simulink model "mult35x35_tb"  (Simulink 6.6)
settings: Solver=ode45  StartTime=0.0  StopTime=1000  RelTol=1e-3
undefined symbols (not defined in the file): A, B
libraries: xbsIndex_r4 x168, simulink x2, xbsCopyrightNotice_r4 x1
(part 1 of 2)
settings Model: Creator=singhj  LastModifiedBy=juttu
settings DataIOCC: SignalLoggingName=sigsOut
settings OptimizationCC: InlineInvariantSignals=on
settings DebuggingCC: SignalResolutionControl=TryResolveAllWithWarning  SolverPrmCheckMsg=none  MultiTaskDSMMsg=warning  MultiTaskCondExecSysMsg=none  StrictBusMsg=None
settings HardwareCC: TargetUnknown=on
settings RTWCC: IncludeERTFirstTime=on

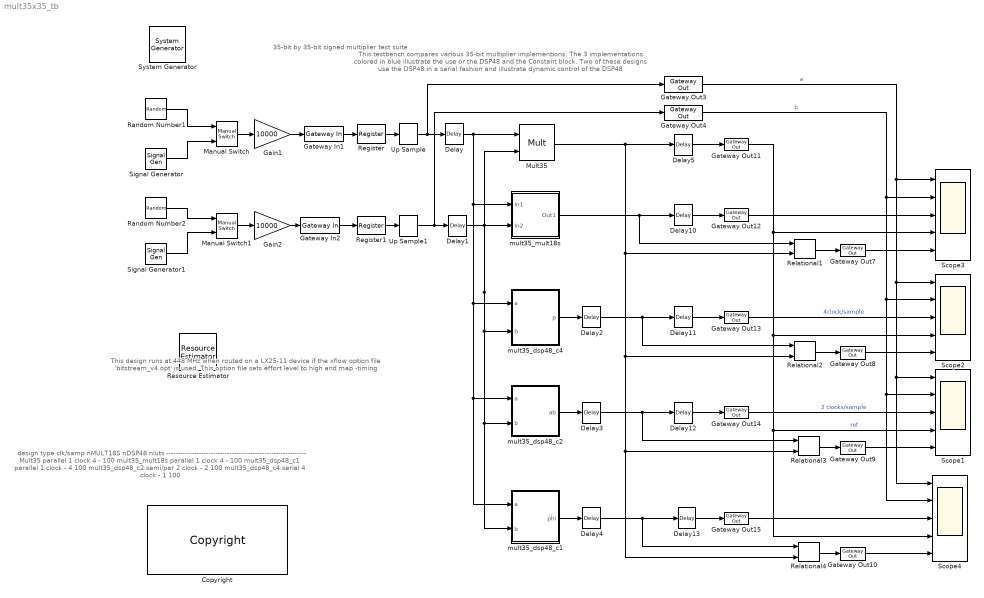
== system mult35x35_tb ==
  note: 35-bit by 35-bit signed multiplier test suite
  note: This testbench compares various 35-bit multiplier implementions.
      | The 3 implementations colored in blue illustrate the use or the DSP48
      | and the Constant block. Two of these designs use the DSP48 in a serial
      | fashion and illustrate dynamic control of the DSP48
  note: design           type       clk/samp  nMULT18S nDSP48 nluts
      | ------------------------------------------------------------
      | Mult35           parallel   1 clock     4       -      100
      | mult35_mult18s   parallel   1 clock     4       -      100
      | mult35_dsp48_c1  parallel   1 clock     -       4      100
      | mult35_dsp48_c2  semi/par   2 clock     -       2      100
      | mult35_dsp48_c4  serial     4 clock     -       1      100
  note: This design runs at 448 MHz
      | when routed on a LX25-11 device if the
      | xflow option file 'bitstream_v4.opt' is used.
      | This option file sets effort level to high
      | and map -timing
  " System Generator" : xbsIndex_r4/ System Generator  Tag=genX  SystemSampleTime=-1  xilinxfamily=Virtex4  part=xc4vlx25  speed=-11  package=ff668  synthesis_tool=Synplify Pro  clock_wrapper=Clock Enables  directory=./netlist  testbench=off  simulink_period=1  sysclk_period=100  dcm_input_clock_period=100  incr_netlist=off  trim_vbits=Everywhere in SubSystem  dbl_ovrd=According to Block Masks  core_generation=According to Block Masks  run_coregen=off  deprecated_control=off  eval_field=0  block_type=sysgen
      settings: block_version=8.2.EA1
  Copyright : xbsCopyrightNotice_r4/Copyright  block_type=copyright
      settings: block_version=10.1.00
      settings: infoedit=|
      | Copyright(C) 2008 by  Xilinx, Inc. All rights reserved.<br>
      | <br>
      | This file contains proprietary, confidential information of Xilinx, Inc., is distributed under license
      | from Xilinx, Inc., and may be used, copied and/or disclosed only pursuant to the terms of a valid license
      | agreement with Xilinx, Inc. Xilinx hereby grants you a license to use this file solely for design,
      | simulation, implementation and creation of design files limited to Xilinx devices or technologies. Use
      | with non-Xilinx devices or technologies is expressly prohibited and immediately terminates your license
      | unless covered by a separate agreement.<br>
      | <br>
      | Xilinx is providing this design, code, or information "as-is" solely for use in developing programs and
      | solutions for Xilinx devices, with no obligation on the part of Xilinx to provide support. By providing
      | this design, code, or information as one possible implementation of this feature, application or standard,
      | Xilinx is making no representation that this implementation is free from any claims of infringement. You
      | are responsible for obtaining any rights you may require for your implementation. Xilinx expressly disclaims
      | any warranty whatsoever with respect to the adequacy of the implementation, including but not limited to any
      | warranties or representations that this implementation is free from claims of infringement, implied warranties
      | of merchantability or fitness for a particular purpose.<br>
      | <br>
      | Xilinx products are not intended for use in life support appliances, devices, or systems. Use in such
      | applications is expressly prohibited.<br>
      | <br>
      | Any modifications that are made to the Source Code are done at the user's sole risk and will be unsupported.<br>
      | <br>
      | This copyright and support notice must be retained as part of this text at all times.
      | (c) Copyright 1995-2008 Xilinx, Inc. All rights reserved.
  Delay{,1..4} (5 alike) : xbsIndex_r4/Delay  en=off  latency=3  dbl_ovrd=off  reg_retiming=on  block_type=delay
      settings: infoedit="Delay line having  configurable length.<P><P>Hardware notes: A delay line is a chain, each link of which is an SRL16 followed by a flip-flop. If register retiming is enabled, the delay line is a chain of flip-flops."  xl_area=[0, 0, 0, 0, 0, 0, 0]  block_version=VER_STRING_GOES_HERE
  Delay10 : xbsIndex_r4/Delay  en=off  latency=15  dbl_ovrd=off  reg_retiming=on  block_type=delay
      settings: infoedit="Delay line having  configurable length.<P><P>Hardware notes: A delay line is a chain, each link of which is an SRL16 followed by a flip-flop. If register retiming is enabled, the delay line is a chain of flip-flops."  xl_area=[0, 0, 0, 0, 0, 0, 0]  block_version=VER_STRING_GOES_HERE
  Delay11 : xbsIndex_r4/Delay  en=off  latency=5  dbl_ovrd=off  reg_retiming=on  block_type=delay
      settings: infoedit="Delay line having  configurable length.<P><P>Hardware notes: A delay line is a chain, each link of which is an SRL16 followed by a flip-flop. If register retiming is enabled, the delay line is a chain of flip-flops."  xl_area=[0, 0, 0, 0, 0, 0, 0]  block_version=VER_STRING_GOES_HERE
  Delay12 : xbsIndex_r4/Delay  en=off  latency=6  dbl_ovrd=off  reg_retiming=on  block_type=delay
      settings: infoedit="Delay line having  configurable length.<P><P>Hardware notes: A delay line is a chain, each link of which is an SRL16 followed by a flip-flop. If register retiming is enabled, the delay line is a chain of flip-flops."  xl_area=[0, 0, 0, 0, 0, 0, 0]  block_version=VER_STRING_GOES_HERE
  Delay13 : xbsIndex_r4/Delay  en=off  latency=9  dbl_ovrd=off  reg_retiming=on  block_type=delay
      settings: infoedit="Delay line having  configurable length.<P><P>Hardware notes: A delay line is a chain, each link of which is an SRL16 followed by a flip-flop. If register retiming is enabled, the delay line is a chain of flip-flops."  xl_area=[0, 0, 0, 0, 0, 0, 0]  block_version=VER_STRING_GOES_HERE
  Delay5 : xbsIndex_r4/Delay  en=off  latency=13  dbl_ovrd=off  reg_retiming=on  block_type=delay
      settings: infoedit="Delay line having  configurable length.<P><P>Hardware notes: A delay line is a chain, each link of which is an SRL16 followed by a flip-flop. If register retiming is enabled, the delay line is a chain of flip-flops."  xl_area=[0, 0, 0, 0, 0, 0, 0]  block_version=VER_STRING_GOES_HERE
  Gain1 : Gain  Gain=10000  SampleTime=4  SaturateOnIntegerOverflow=on
  Gain2 : Gain  Gain=10000  SampleTime=4  SaturateOnIntegerOverflow=on
  Gateway In1 : xbsIndex_r4/Gateway In  arith_type="Signed  (2's comp)"  n_bits=35  bin_pt=0  quantization="Round  (unbiased: +/- Inf)"  overflow=Saturate  period=4  dbl_ovrd=off  timing_constraint=None  locs_specified=off  LOCs={}  block_type=gatewayin
      settings: infoedit="Gateway in block.  Converts inputs of type Simulink integer, double and fixed point to  Xilinx fixed point type.<P><P>Hardware notes:  In hardware these blocks become top level input ports."  xl_area=[0 0 0 0 35 0 0]  block_version=VER_STRING_GOES_HERE
  Gateway In2 : xbsIndex_r4/Gateway In  arith_type="Signed  (2's comp)"  n_bits=35  bin_pt=0  quantization="Round  (unbiased: +/- Inf)"  overflow=Saturate  period=4  dbl_ovrd=off  timing_constraint=None  locs_specified=off  LOCs={}  block_type=gatewayin
      settings: infoedit="Gateway in block.  Converts inputs of type Simulink integer, double and fixed point to  Xilinx fixed point type.<P><P>Hardware notes:  In hardware these blocks become top level input ports."  xl_area=[0 0 0 0 35 0 0]  block_version=VER_STRING_GOES_HERE
  Gateway Out{7..15} (9 alike) : xbsIndex_r4/Gateway Out  hdl_port=on  timing_constraint=None  locs_specified=off  LOCs={}  block_type=gatewayout
      settings: infoedit="Gateway out block.  Converts Xilinx fixed point inputs into ouputs of type Simulink integer, double, or fixed point.<P><P>Hardware notes:  In hardware these blocks become top level output ports or are discarded, depending on how they are configured."  xl_area=[0 0 0 0 70 0 0]  block_version=VER_STRING_GOES_HERE
  Gateway Out3 : xbsIndex_r4/Gateway Out  hdl_port=off  timing_constraint=None  locs_specified=off  LOCs={}  block_type=gatewayout
      settings: infoedit="Gateway out block.  Converts Xilinx fixed point inputs into ouputs of type Simulink integer, double, or fixed point.<P><P>Hardware notes:  In hardware these blocks become top level output ports or are discarded, depending on how they are configured."  xl_area=[0 0 0 0 70 0 0]  block_version=VER_STRING_GOES_HERE
  Gateway Out4 : xbsIndex_r4/Gateway Out  hdl_port=off  timing_constraint=None  locs_specified=off  LOCs={}  block_type=gatewayout
      settings: infoedit="Gateway out block.  Converts Xilinx fixed point inputs into ouputs of type Simulink integer, double, or fixed point.<P><P>Hardware notes:  In hardware these blocks become top level output ports or are discarded, depending on how they are configured."  xl_area=[0 0 0 0 70 0 0]  block_version=VER_STRING_GOES_HERE
  Manual Switch : simulink/Signal Routing/Manual Switch  SystemSampleTime=-1  sw=0  action=0  varsize=off
  Manual Switch1 : simulink/Signal Routing/Manual Switch  SystemSampleTime=-1  sw=0  action=0  varsize=off
  Mult35 : xbsIndex_r4/Mult  precision=Full  arith_type="Signed  (2's comp)"  n_bits=8  bin_pt=2  quantization=Truncate  overflow=Wrap  en=off  latency=5  dbl_ovrd=off  use_behavioral_HDL=off  use_embedded=on  opt=Speed  optimum_pipeline=off  pipeline=on  use_rpm=on  placement_style=Rectangular shape  block_type=mult
      settings: infoedit=Multiplies two values.<P><P>Hardware notes: To use the internal pipeline stage of the dedicated multiplier you must select 'Pipeline to Greatest Extent Possible'.  xl_area=[231 460 0 269 0 4 0]  block_version=VER_STRING_GOES_HERE
  Random Number1 : RandomNumber  SampleTime=0
  Random Number2 : RandomNumber  SampleTime=0
  Register : xbsIndex_r4/Register  init=0  rst=off  en=off  dbl_ovrd=off  block_type=register
      settings: block_version=VER_STRING_GOES_HERE
  Register1 : xbsIndex_r4/Register  init=0  rst=off  en=off  dbl_ovrd=off  block_type=register
      settings: block_version=VER_STRING_GOES_HERE
  Relational{1..4} (4 alike) : xbsIndex_r4/Relational  mode=a!=b  en=off  latency=1  dbl_ovrd=off  block_type=relational
      settings: block_version=10.1.2-Beta
  Resource Estimator : xbsIndex_r4/Resource Estimator  Tag=resEstTag  Slices=896  FFs=1554  BRAMs=0  LUTs=775  IOBs=545  EBMs=8  TBUFs=0  xl_use_estimator_area=off  est_options=Estimate  xl_estimator_area=[896 1554 0 775 545 8 0]  mrp_directory=C:/1proj/designs/firs/fir_t1_pipe/par_v1_g1  simulink_period=1/16  block_type=resource_estimator
      settings: AttributesFormatString=Resource\nEstimator  block_version=8.2.EA1
  Scope{1..4} (4 alike) : Scope  NumInputPorts=5
      Scope1 settings: TimeRange=100  YMin=-100~-100~0~0~-1  YMax=100~100~10000~10000~1
      Scope2 settings: TimeRange=100  YMin=-100~-100~0~0~-1  YMax=100~100~10000~10000~1  SaveName=ScopeData3
      Scope3 settings: TimeRange=100  YMin=-100~-100~0~0~-1  YMax=100~100~10000~10000~1  SaveName=ScopeData4
      Scope4 settings: TimeRange=100  YMin=-100~-100~0~0~-1  YMax=100~100~10000~10000~1  SaveName=ScopeData5
  Signal Generator : SignalGenerator  Amplitude=100  Frequency=.00300
  Signal Generator1 : SignalGenerator  Amplitude=100  Frequency=.0200
  Up Sample : xbsIndex_r4/Up Sample  sample_ratio=4  copy_samples=on  dbl_ovrd=off  block_type=usamp
      settings: infoedit="Up samples input data.  Inserted values  can be zeros or copies of the most recent input sample.<P><P>Hardware notes: No hardware is needed if inserted values are copies of the input sample; otherwise, a mux and single bit flip-flop are used."  xl_area=[0, 0, 0, 0, 0, 0, 0]  block_version=VER_STRING_GOES_HERE
  Up Sample1 : xbsIndex_r4/Up Sample  sample_ratio=4  copy_samples=on  dbl_ovrd=off  block_type=usamp
      settings: infoedit="Up samples input data.  Inserted values  can be zeros or copies of the most recent input sample.<P><P>Hardware notes: No hardware is needed if inserted values are copies of the input sample; otherwise, a mux and single bit flip-flop are used."  xl_area=[0, 0, 0, 0, 0, 0, 0]  block_version=VER_STRING_GOES_HERE
  mult35_dsp48_c1 : Subsystem
  mult35_dsp48_c2 : Subsystem
  mult35_dsp48_c4 : Subsystem
  mult35_mult18s : Subsystem
  wires:
  Mult35/1 -> Relational1/2, Relational2/2, Relational3/2, Relational4/2, Delay5/1
  mult35_dsp48_c4/1(p) -> Delay2/1
  mult35_mult18s/1(Out1) -> Relational1/1, Delay10/1
  Signal Generator/1 -> Manual Switch/2
  mult35_dsp48_c2/1(ab) -> Delay3/1
  mult35_dsp48_c1/1(phi) -> Delay4/1
  Random Number1/1 -> Manual Switch/1
  Manual Switch/1 -> Gain1/1
  Gain1/1 -> Gateway In1/1
  Signal Generator1/1 -> Manual Switch1/2
  Random Number2/1 -> Manual Switch1/1
  Manual Switch1/1 -> Gain2/1
  Gateway In1/1 -> Register/1
  Gateway In2/1 -> Register1/1
  Gateway Out11/1 -> Scope3/4, Scope2/4, Scope1/4, Scope4/4  "ref"
  Gateway Out14/1 -> Scope1/3  "2 clocks/sample"
  Gateway Out13/1 -> Scope2/3  "4clock/sample"
  Gateway Out12/1 -> Scope3/3
  Gain2/1 -> Gateway In2/1
  Delay/1 -> mult35_dsp48_c1/1(a), mult35_dsp48_c2/1(a), mult35_dsp48_c4/1(a), mult35_mult18s/1(In1), Mult35/1
  Delay1/1 -> mult35_dsp48_c1/2(b), mult35_dsp48_c2/2(b), mult35_dsp48_c4/2(b), mult35_mult18s/2(In2), Mult35/2
  Delay2/1 -> Relational2/1, Delay11/1
  Delay3/1 -> Relational3/1, Delay12/1
  Delay4/1 -> Relational4/1, Delay13/1
  Up Sample/1 -> Delay/1, Gateway Out3/1
  Up Sample1/1 -> Delay1/1, Gateway Out4/1
  Gateway Out3/1 -> Scope3/1, Scope2/1, Scope4/1, Scope1/1  "a"
  Gateway Out4/1 -> Scope4/2, Scope1/2, Scope2/2, Scope3/2  "b"
  Gateway Out15/1 -> Scope4/3
  Register/1 -> Up Sample/1
  Register1/1 -> Up Sample1/1
  Relational1/1 -> Gateway Out7/1
  Gateway Out8/1 -> Scope2/5
  Gateway Out9/1 -> Scope1/5
  Gateway Out7/1 -> Scope3/5
  Relational2/1 -> Gateway Out8/1
  Relational3/1 -> Gateway Out9/1
  Relational4/1 -> Gateway Out10/1
  Gateway Out10/1 -> Scope4/5
  Delay5/1 -> Gateway Out11/1
  Delay10/1 -> Gateway Out12/1
  Delay11/1 -> Gateway Out13/1
  Delay12/1 -> Gateway Out14/1
  Delay13/1 -> Gateway Out15/1

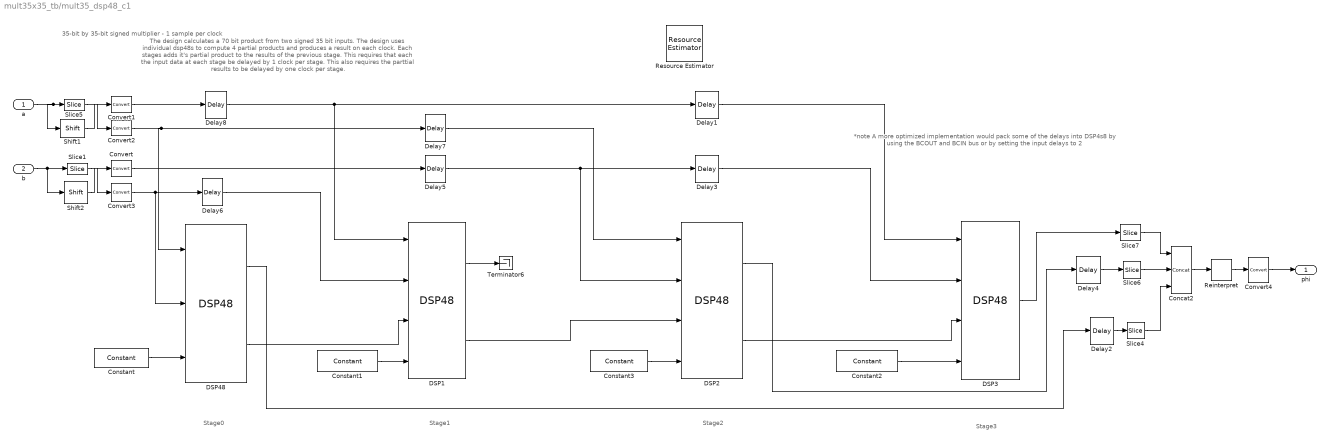
== system mult35x35_tb/mult35_dsp48_c1 ==
  note: The design calculates a 70 bit product from two signed 35 bit inputs.
      | The design uses individual dsp48s to compute 4 partial products and produces a result on each clock.
      | Each stages adds it's partial product to the results of the previous stage. This requires that each the
      | input data at each stage be delayed by 1 clock per stage. This also requires the parttial results to be delayed
      | by one clock per stage.
  note: 35-bit by 35-bit signed multiplier -
      | 1 sample per clock
  note: *note
      | A more optimized implementation
      | would pack some of the delays into
      | DSP4s8 by using the BCOUT and BCIN
      |  bus or  by setting the input delays to 2
  note: Stage3
  note: Stage2
  note: Stage1
  note: Stage0
  a : Inport
  b : Inport  Port=2
  Concat2 : xbsIndex_r4/Concat  num_inputs=3  dbl_ovrd=off  block_type=concat
      settings: block_version=VER_STRING_GOES_HERE
  Constant : xbsIndex_r4/Constant  arith_type=DSP48 Instruction  const=1  n_bits=1  bin_pt=0  explicit_period=off  period=1  equ=P=+A*B  opselect=A * B  inp2=PCIN>>17  opr=+  inp1=P  carry=CIN  dbl_ovrd=off  block_type=constant
      settings: block_version=VER_STRING_GOES_HERE
  Constant1 : xbsIndex_r4/Constant  arith_type=DSP48 Instruction  const=1  n_bits=1  bin_pt=0  explicit_period=off  period=1  equ=P=PCIN>>17+(A*B)  opselect=Custom  inp2=PCIN>>17  opr=+  inp1=A*B  carry=0  dbl_ovrd=off  block_type=constant
      settings: block_version=VER_STRING_GOES_HERE
  Constant2 : xbsIndex_r4/Constant  arith_type=DSP48 Instruction  const=1  n_bits=1  bin_pt=0  explicit_period=off  period=1  equ=P=PCIN>>17+(A*B)  opselect=Custom  inp2=PCIN>>17  opr=+  inp1=A*B  carry=0  dbl_ovrd=off  block_type=constant
      settings: block_version=VER_STRING_GOES_HERE
  Constant3 : xbsIndex_r4/Constant  arith_type=DSP48 Instruction  const=1  n_bits=1  bin_pt=0  explicit_period=off  period=1  equ=P=PCIN+(A*B)  opselect=Custom  inp2=PCIN  opr=+  inp1=A*B  carry=0  dbl_ovrd=off  block_type=constant
      settings: block_version=VER_STRING_GOES_HERE
  Convert{,1..3} (4 alike) : xbsIndex_r4/Convert  arith_type="Signed  (2's comp)"  n_bits=18  bin_pt=0  quantization=Truncate  overflow=Wrap  latency=0  dbl_ovrd=off  pipeline=off  block_type=convert
      settings: infoedit=The input is presented at the output after quantization and overflow effects.<P><P>Hardware notes: Additional hardware is used when rounding or saturation is selected and output width is less than the input width.  xl_area=[0 0 0 0 0 0 0]  block_version=VER_STRING_GOES_HERE
  Convert4 : xbsIndex_r4/Convert  arith_type="Signed  (2's comp)"  n_bits=71  bin_pt=0  quantization=Truncate  overflow=Wrap  latency=0  dbl_ovrd=off  pipeline=off  block_type=convert
      settings: infoedit=The input is presented at the output after quantization and overflow effects.<P><P>Hardware notes: Additional hardware is used when rounding or saturation is selected and output width is less than the input width.  xl_area=[0 0 0 0 0 0 0]  block_version=VER_STRING_GOES_HERE
  DSP1 : xbsIndex_r4/DSP48  use_b=Direct from B Port  use_op=on  use_creg=off  use_pcin=on  use_pcout=on  use_bcout=off  rst_all=off  en_all=off  pipeline_a=1  pipeline_b=1  pipeline_c=on  pipeline_p=on  pipeline_mult=on  pipeline_opmode=on  pipeline_sub=on  pipeline_carryin=on  pipeline_carryinsel=on  rst_a=off  rst_b=off  rst_c=off  rst_mult=off  rst_p=off  rst_carry_in=off  rst_ctrl=off  en_a=off  en_b=off  en_c=off  en_mult=off  en_p=off  en_carry_in=off  en_ctrl=off  dbl_ovrd=off  use_synth_model=off  xl_useadderonly=off  block_type=dsp48
      settings: xl_use_area=on  xl_area=[0, 0, 0, 0, 0, 0, 0]  block_version=VER_STRING_GOES_HERE
  DSP2 : xbsIndex_r4/DSP48  use_b=Direct from B Port  use_op=on  use_creg=off  use_pcin=on  use_pcout=on  use_bcout=off  rst_all=off  en_all=off  pipeline_a=1  pipeline_b=1  pipeline_c=on  pipeline_p=on  pipeline_mult=on  pipeline_opmode=on  pipeline_sub=on  pipeline_carryin=on  pipeline_carryinsel=on  rst_a=off  rst_b=off  rst_c=off  rst_mult=off  rst_p=off  rst_carry_in=off  rst_ctrl=off  en_a=off  en_b=off  en_c=off  en_mult=off  en_p=off  en_carry_in=off  en_ctrl=off  dbl_ovrd=off  use_synth_model=off  xl_useadderonly=off  block_type=dsp48
      settings: xl_use_area=on  xl_area=[0, 0, 0, 0, 0, 0, 0]  block_version=VER_STRING_GOES_HERE
  DSP3 : xbsIndex_r4/DSP48  use_b=Direct from B Port  use_op=on  use_creg=off  use_pcin=on  use_pcout=off  use_bcout=off  rst_all=off  en_all=off  pipeline_a=1  pipeline_b=1  pipeline_c=on  pipeline_p=on  pipeline_mult=on  pipeline_opmode=on  pipeline_sub=on  pipeline_carryin=on  pipeline_carryinsel=on  rst_a=off  rst_b=off  rst_c=off  rst_mult=off  rst_p=off  rst_carry_in=off  rst_ctrl=off  en_a=off  en_b=off  en_c=off  en_mult=off  en_p=off  en_carry_in=off  en_ctrl=off  dbl_ovrd=off  use_synth_model=off  xl_useadderonly=off  block_type=dsp48
      settings: xl_use_area=on  xl_area=[0, 0, 0, 0, 0, 0, 0]  block_version=VER_STRING_GOES_HERE
  DSP48 : xbsIndex_r4/DSP48  use_b=Direct from B Port  use_op=on  use_creg=off  use_pcin=off  use_pcout=on  use_bcout=off  rst_all=off  en_all=off  pipeline_a=1  pipeline_b=1  pipeline_c=on  pipeline_p=on  pipeline_mult=on  pipeline_opmode=on  pipeline_sub=on  pipeline_carryin=on  pipeline_carryinsel=on  rst_a=off  rst_b=off  rst_c=off  rst_mult=off  rst_p=off  rst_carry_in=off  rst_ctrl=off  en_a=off  en_b=off  en_c=off  en_mult=off  en_p=off  en_carry_in=off  en_ctrl=off  dbl_ovrd=off  use_synth_model=off  xl_useadderonly=off  block_type=dsp48
      settings: xl_use_area=on  xl_area=[0, 0, 0, 0, 0, 0, 0]  block_version=VER_STRING_GOES_HERE
  Delay1 : xbsIndex_r4/Delay  en=off  latency=2  dbl_ovrd=off  reg_retiming=off  block_type=delay
      settings: infoedit="Delay line having  configurable length.<P><P>Hardware notes: A delay line is a chain, each link of which is an SRL16 followed by a flip-flop. If register retiming is enabled, the delay line is a chain of flip-flops."  xl_area=[9 18 0 18 0 0 0]  block_version=VER_STRING_GOES_HERE
  Delay2 : xbsIndex_r4/Delay  en=off  latency=3  dbl_ovrd=off  reg_retiming=off  block_type=delay
      settings: infoedit="Delay line having  configurable length.<P><P>Hardware notes: A delay line is a chain, each link of which is an SRL16 followed by a flip-flop. If register retiming is enabled, the delay line is a chain of flip-flops."  xl_area=[24 48 0 48 0 0 0]  block_version=VER_STRING_GOES_HERE
  Delay{3..4,6,8} (4 alike) : xbsIndex_r4/Delay  en=off  latency=1  dbl_ovrd=off  reg_retiming=off  block_type=delay
      Delay3 settings: infoedit="Delay line having  configurable length.<P><P>Hardware notes: A delay line is a chain, each link of which is an SRL16 followed by a flip-flop. If register retiming is enabled, the delay line is a chain of flip-flops."  xl_area=[9 18 0 0 0 0 0]  block_version=VER_STRING_GOES_HERE
      Delay4 settings: infoedit="Delay line having  configurable length.<P><P>Hardware notes: A delay line is a chain, each link of which is an SRL16 followed by a flip-flop. If register retiming is enabled, the delay line is a chain of flip-flops."  xl_area=[24 48 0 0 0 0 0]  block_version=VER_STRING_GOES_HERE
      Delay6 settings: infoedit="Delay line having  configurable length.<P><P>Hardware notes: A delay line is a chain, each link of which is an SRL16 followed by a flip-flop. If register retiming is enabled, the delay line is a chain of flip-flops."  xl_area=[9 18 0 0 0 0 0]  block_version=VER_STRING_GOES_HERE
      Delay8 settings: infoedit="Delay line having  configurable length.<P><P>Hardware notes: A delay line is a chain, each link of which is an SRL16 followed by a flip-flop. If register retiming is enabled, the delay line is a chain of flip-flops."  xl_area=[9 18 0 0 0 0 0]  block_version=VER_STRING_GOES_HERE
  Delay5 : xbsIndex_r4/Delay  en=off  latency=2  dbl_ovrd=off  reg_retiming=off  block_type=delay
      settings: infoedit="Delay line having  configurable length.<P><P>Hardware notes: A delay line is a chain, each link of which is an SRL16 followed by a flip-flop. If register retiming is enabled, the delay line is a chain of flip-flops."  xl_area=[9 18 0 18 0 0 0]  block_version=VER_STRING_GOES_HERE
  Delay7 : xbsIndex_r4/Delay  en=off  latency=2  dbl_ovrd=off  reg_retiming=off  block_type=delay
      settings: infoedit="Delay line having  configurable length.<P><P>Hardware notes: A delay line is a chain, each link of which is an SRL16 followed by a flip-flop. If register retiming is enabled, the delay line is a chain of flip-flops."  xl_area=[9 18 0 18 0 0 0]  block_version=VER_STRING_GOES_HERE
  Reinterpret : xbsIndex_r4/Reinterpret  force_arith_type=on  arith_type="Signed  (2's comp)"  force_bin_pt=on  bin_pt=0  block_type=cast
      settings: infoedit="Changes type of samples without altering their binary representation.<P><P>Hardware notes: In hardware this block costs nothing.<P><P>Example:  Suppose the input is 6 bits wide, signed, with 2 fractional bits, and the output is forced to unsigned with 0 fractional bits.  Then an input of -2.0 (1110.00 in binary 2's complement) becomes an output of 56 (111000 in binary)."  block_version=VER_STRING_GOES_HERE
  Resource Estimator : xbsIndex_r4/Resource Estimator  Tag=resEstTag  Slices=102  FFs=204  BRAMs=0  LUTs=102  IOBs=0  EBMs=0  TBUFs=0  xl_use_estimator_area=off  est_options=Estimate  xl_estimator_area=[102 204 0 102 0 0 0]  mrp_directory=I:\sg48\src  simulink_period=1/16  block_type=resource_estimator
      settings: AttributesFormatString=Resource\nEstimator  block_version=9.2.00
  Shift1 : xbsIndex_r4/Shift  shift_dir=Right  shift_bits=17  en=off  latency=0  precision=Full  arith_type="Signed  (2's comp)"  n_bits=8  bin_pt=2  quantization=Truncate  overflow=Wrap  dbl_ovrd=off  block_type=shift
      settings: xl_area=[0 0 0 0 0 0 0]  block_version=VER_STRING_GOES_HERE
  Shift2 : xbsIndex_r4/Shift  shift_dir=Right  shift_bits=17  en=off  latency=0  precision=Full  arith_type="Signed  (2's comp)"  n_bits=8  bin_pt=2  quantization=Truncate  overflow=Wrap  dbl_ovrd=off  block_type=shift
      settings: xl_area=[0 0 0 0 0 0 0]  block_version=VER_STRING_GOES_HERE
  Slice{1,4..6} (4 alike) : xbsIndex_r4/Slice  nbits=17  boolean_output=off  mode=Lower Bit Location + Width  bit1=18  base1=LSB of Input  bit0=0  base0=LSB of Input  dbl_ovrd=off  block_type=slice
      settings: infoedit="Extracts a given range of bits from each input sample and presents it at the output.  The output type is ordinarily unsigned with binary point at zero, but can be Boolean when the slice is one bit wide.<P><P>Hardware notes: In hardware this block costs nothing."  block_version=VER_STRING_GOES_HERE
  Slice7 : xbsIndex_r4/Slice  nbits=36  boolean_output=off  mode=Lower Bit Location + Width  bit1=18  base1=LSB of Input  bit0=0  base0=LSB of Input  dbl_ovrd=off  block_type=slice
      settings: infoedit="Extracts a given range of bits from each input sample and presents it at the output.  The output type is ordinarily unsigned with binary point at zero, but can be Boolean when the slice is one bit wide.<P><P>Hardware notes: In hardware this block costs nothing."  block_version=VER_STRING_GOES_HERE
  Terminator6 : Terminator
  phi : Outport
  wires:
  Convert4/1 -> phi/1
  Slice4/1 -> Concat2/3
  Slice6/1 -> Concat2/2
  Delay2/1 -> Slice4/1
  Slice7/1 -> Concat2/1
  Delay4/1 -> Slice6/1
  DSP3/1 -> Slice7/1
  Reinterpret/1 -> Convert4/1
  Concat2/1 -> Reinterpret/1
  Convert3/1 -> Delay6/1, DSP48/2
  Convert/1 -> Delay5/1
  Convert2/1 -> Delay7/1, DSP48/1
  Convert1/1 -> Delay8/1
  Delay1/1 -> DSP3/1
  Delay3/1 -> DSP3/2
  Delay7/1 -> DSP2/1
  Delay5/1 -> Delay3/1, DSP2/2
  Constant3/1 -> DSP2/4
  Delay8/1 -> Delay1/1, DSP1/1
  b/1 -> Shift2/1, Slice1/1
  a/1 -> Shift1/1, Slice5/1
  Delay6/1 -> DSP1/2
  Constant1/1 -> DSP1/4
  Constant/1 -> DSP48/3
  Constant2/1 -> DSP3/4
  Shift2/1 -> Convert/1
  Slice1/1 -> Convert3/1
  Shift1/1 -> Convert1/1
  Slice5/1 -> Convert2/1
  DSP48/1 -> Delay2/1
  DSP2/1 -> Delay4/1
  DSP48/2 -> DSP1/3
  DSP2/2 -> DSP3/3
  DSP1/1 -> Terminator6/1
  DSP1/2 -> DSP2/3

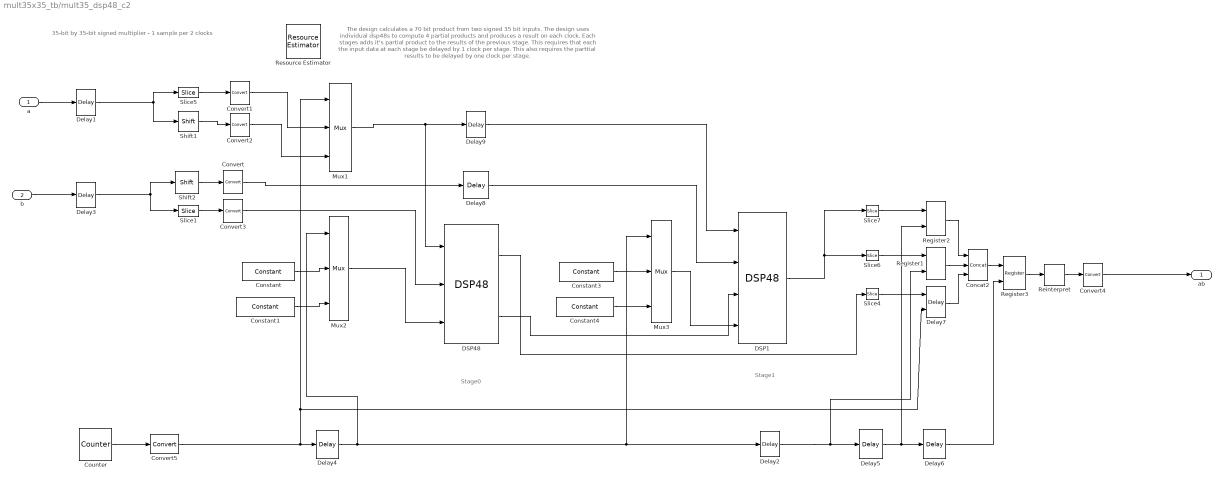
== system mult35x35_tb/mult35_dsp48_c2 ==
  note: 35-bit by 35-bit signed multiplier -
      | 1 sample per 2 clocks
  note: The design calculates a 70 bit product from two signed 35 bit inputs.
      | The design uses individual dsp48s to compute 4 partial products and produces a result on each clock.
      | Each stages adds it's partial product to the results of the previous stage. This requires that each the
      | input data at each stage be delayed by 1 clock per stage. This also requires the parttial results to be delayed
      | by one clock per stage.
  note: Stage0
  note: Stage1
  a : Inport
  b : Inport  Port=2
  Concat2 : xbsIndex_r4/Concat  num_inputs=3  dbl_ovrd=off  block_type=concat
      settings: block_version=VER_STRING_GOES_HERE
  Constant : xbsIndex_r4/Constant  arith_type=DSP48 Instruction  const=1  n_bits=1  bin_pt=0  explicit_period=off  period=1  equ=P=+A*B  opselect=A * B  inp2=PCIN>>17  opr=+  inp1=P  carry=CIN  dbl_ovrd=off  block_type=constant
      settings: block_version=VER_STRING_GOES_HERE
  Constant1 : xbsIndex_r4/Constant  arith_type=DSP48 Instruction  const=1  n_bits=1  bin_pt=0  explicit_period=off  period=1  equ=P=P>>17+(A*B)  opselect=Custom  inp2=P>>17  opr=+  inp1=A*B  carry=0  dbl_ovrd=off  block_type=constant
      settings: block_version=VER_STRING_GOES_HERE
  Constant3 : xbsIndex_r4/Constant  arith_type=DSP48 Instruction  const=1  n_bits=1  bin_pt=0  explicit_period=off  period=1  equ=P=PCIN+(A*B)  opselect=Custom  inp2=PCIN  opr=+  inp1=A*B  carry=0  dbl_ovrd=off  block_type=constant
      settings: block_version=VER_STRING_GOES_HERE
  Constant4 : xbsIndex_r4/Constant  arith_type=DSP48 Instruction  const=1  n_bits=1  bin_pt=0  explicit_period=off  period=1  equ=P=P>>17+(A*B)  opselect=Custom  inp2=P>>17  opr=+  inp1=A*B  carry=0  dbl_ovrd=off  block_type=constant
      settings: block_version=VER_STRING_GOES_HERE
  Convert{,1..3} (4 alike) : xbsIndex_r4/Convert  arith_type="Signed  (2's comp)"  n_bits=18  bin_pt=0  quantization=Truncate  overflow=Wrap  latency=0  dbl_ovrd=off  pipeline=off  block_type=convert
      settings: infoedit=The input is presented at the output after quantization and overflow effects.<P><P>Hardware notes: Additional hardware is used when rounding or saturation is selected and output width is less than the input width.  xl_area=[0 0 0 0 0 0 0]  block_version=VER_STRING_GOES_HERE
  Convert4 : xbsIndex_r4/Convert  arith_type="Signed  (2's comp)"  n_bits=71  bin_pt=0  quantization=Truncate  overflow=Wrap  latency=0  dbl_ovrd=off  pipeline=off  block_type=convert
      settings: infoedit=The input is presented at the output after quantization and overflow effects.<P><P>Hardware notes: Additional hardware is used when rounding or saturation is selected and output width is less than the input width.  xl_area=[0 0 0 0 0 0 0]  block_version=VER_STRING_GOES_HERE
  Convert5 : xbsIndex_r4/Convert  arith_type=Boolean  n_bits=8  bin_pt=6  quantization=Truncate  overflow=Wrap  latency=0  dbl_ovrd=off  pipeline=off  block_type=convert
      settings: infoedit=The input is presented at the output after quantization and overflow effects.<P><P>Hardware notes: Additional hardware is used when rounding or saturation is selected and output width is less than the input width.  xl_area=[0 0 0 0 0 0 0]  block_version=VER_STRING_GOES_HERE
  Counter : xbsIndex_r4/Counter  cnt_type=Free Running  cnt_to=Inf  operation=Up  start_count=0  cnt_by_val=1  arith_type=Unsigned  n_bits=1  bin_pt=0  load_pin=off  rst=off  en=off  explicit_period=off  period=1  dbl_ovrd=off  use_behavioral_HDL=off  use_rpm=off  block_type=counter
      settings: infoedit="Configurable up, down and up/down counter.<P><P>Hardware notes: Free running counters are the least expensive in hardware.  A count limited counter is implemented by combining a counter with a comparator."  xl_area=[1 1 0 1 0 0 0]  block_version=VER_STRING_GOES_HERE
  DSP1 : xbsIndex_r4/DSP48  use_b=Direct from B Port  use_op=on  use_creg=off  use_pcin=on  use_pcout=off  use_bcout=off  rst_all=off  en_all=off  pipeline_a=1  pipeline_b=1  pipeline_c=on  pipeline_p=on  pipeline_mult=on  pipeline_opmode=on  pipeline_sub=on  pipeline_carryin=on  pipeline_carryinsel=on  rst_a=off  rst_b=off  rst_c=off  rst_mult=off  rst_p=off  rst_carry_in=off  rst_ctrl=off  en_a=off  en_b=off  en_c=off  en_mult=off  en_p=off  en_carry_in=off  en_ctrl=off  dbl_ovrd=off  use_synth_model=off  xl_useadderonly=off  block_type=dsp48
      settings: xl_use_area=on  xl_area=[0, 0, 0, 0, 0, 0, 0]  block_version=VER_STRING_GOES_HERE
  DSP48 : xbsIndex_r4/DSP48  use_b=Direct from B Port  use_op=on  use_creg=off  use_pcin=off  use_pcout=on  use_bcout=off  rst_all=off  en_all=off  pipeline_a=1  pipeline_b=1  pipeline_c=on  pipeline_p=on  pipeline_mult=on  pipeline_opmode=on  pipeline_sub=on  pipeline_carryin=on  pipeline_carryinsel=on  rst_a=off  rst_b=off  rst_c=off  rst_mult=off  rst_p=off  rst_carry_in=off  rst_ctrl=off  en_a=off  en_b=off  en_c=off  en_mult=off  en_p=off  en_carry_in=off  en_ctrl=off  dbl_ovrd=off  use_synth_model=off  xl_useadderonly=off  block_type=dsp48
      settings: xl_use_area=on  xl_area=[0, 0, 0, 0, 0, 0, 0]  block_version=VER_STRING_GOES_HERE
  Delay1 : xbsIndex_r4/Delay  en=off  latency=1  dbl_ovrd=off  reg_retiming=on  block_type=delay
      settings: infoedit="Delay line having  configurable length.<P><P>Hardware notes: A delay line is a chain, each link of which is an SRL16 followed by a flip-flop. If register retiming is enabled, the delay line is a chain of flip-flops."  xl_area=[9 18 0 18 0 0 0]  block_version=VER_STRING_GOES_HERE
  Delay{2..6} (5 alike) : xbsIndex_r4/Delay  en=off  latency=1  dbl_ovrd=off  reg_retiming=off  block_type=delay
      Delay2 settings: infoedit="Delay line having  configurable length.<P><P>Hardware notes: A delay line is a chain, each link of which is an SRL16 followed by a flip-flop. If register retiming is enabled, the delay line is a chain of flip-flops."  xl_area=[1 1 0 0 0 0 0]  block_version=VER_STRING_GOES_HERE
      Delay3 settings: infoedit="Delay line having  configurable length.<P><P>Hardware notes: A delay line is a chain, each link of which is an SRL16 followed by a flip-flop. If register retiming is enabled, the delay line is a chain of flip-flops."  xl_area=[9 18 0 18 0 0 0]  block_version=VER_STRING_GOES_HERE
      Delay4 settings: infoedit="Delay line having  configurable length.<P><P>Hardware notes: A delay line is a chain, each link of which is an SRL16 followed by a flip-flop. If register retiming is enabled, the delay line is a chain of flip-flops."  xl_area=[1 1 0 0 0 0 0]  block_version=VER_STRING_GOES_HERE
      Delay5 settings: infoedit="Delay line having  configurable length.<P><P>Hardware notes: A delay line is a chain, each link of which is an SRL16 followed by a flip-flop. If register retiming is enabled, the delay line is a chain of flip-flops."  xl_area=[1 1 0 0 0 0 0]  block_version=VER_STRING_GOES_HERE
      Delay6 settings: infoedit="Delay line having  configurable length.<P><P>Hardware notes: A delay line is a chain, each link of which is an SRL16 followed by a flip-flop. If register retiming is enabled, the delay line is a chain of flip-flops."  xl_area=[1 1 0 0 0 0 0]  block_version=VER_STRING_GOES_HERE
  Delay7 : xbsIndex_r4/Delay  en=on  latency=2  dbl_ovrd=off  reg_retiming=off  block_type=delay
      settings: infoedit="Delay line having  configurable length.<P><P>Hardware notes: A delay line is a chain, each link of which is an SRL16 followed by a flip-flop. If register retiming is enabled, the delay line is a chain of flip-flops."  xl_area=[9 17 0 17 0 0 0]  block_version=VER_STRING_GOES_HERE
  Delay8 : xbsIndex_r4/Delay  en=off  latency=2  dbl_ovrd=off  reg_retiming=off  block_type=delay
      settings: infoedit="Delay line having  configurable length.<P><P>Hardware notes: A delay line is a chain, each link of which is an SRL16 followed by a flip-flop. If register retiming is enabled, the delay line is a chain of flip-flops."  xl_area=[9 18 0 18 0 0 0]  block_version=VER_STRING_GOES_HERE
  Delay9 : xbsIndex_r4/Delay  en=off  latency=2  dbl_ovrd=off  reg_retiming=off  block_type=delay
      settings: infoedit="Delay line having  configurable length.<P><P>Hardware notes: A delay line is a chain, each link of which is an SRL16 followed by a flip-flop. If register retiming is enabled, the delay line is a chain of flip-flops."  xl_area=[9 18 0 18 0 0 0]  block_version=VER_STRING_GOES_HERE
  Mux1 : xbsIndex_r4/Mux  inputs=2  en=off  latency=0  precision=Full  arith_type=Unsigned  n_bits=48  bin_pt=0  quantization=Truncate  overflow=Wrap  dbl_ovrd=off  block_type=mux
      settings: xl_area=[9 0 0 18 0 0 0]  block_version=VER_STRING_GOES_HERE
  Mux2 : xbsIndex_r4/Mux  inputs=2  en=off  latency=0  precision=Full  arith_type=Unsigned  n_bits=48  bin_pt=0  quantization=Truncate  overflow=Wrap  dbl_ovrd=off  block_type=mux
      settings: xl_area=[6 0 0 11 0 0 0]  block_version=VER_STRING_GOES_HERE
  Mux3 : xbsIndex_r4/Mux  inputs=2  en=off  latency=0  precision=Full  arith_type=Unsigned  n_bits=48  bin_pt=0  quantization=Truncate  overflow=Wrap  dbl_ovrd=off  block_type=mux
      settings: xl_area=[6 0 0 11 0 0 0]  block_version=VER_STRING_GOES_HERE
  Register1 : xbsIndex_r4/Register  init=0  rst=off  en=on  dbl_ovrd=off  block_type=register
      settings: xl_area=[9 17 0 0 0 0 0]  block_version=VER_STRING_GOES_HERE
  Register2 : xbsIndex_r4/Register  init=0  rst=off  en=on  dbl_ovrd=off  block_type=register
      settings: xl_area=[18 36 0 0 0 0 0]  block_version=VER_STRING_GOES_HERE
  Register3 : xbsIndex_r4/Register  init=0  rst=off  en=on  dbl_ovrd=off  block_type=register
      settings: xl_area=[35 70 0 0 0 0 0]  block_version=VER_STRING_GOES_HERE
  Reinterpret : xbsIndex_r4/Reinterpret  force_arith_type=on  arith_type="Signed  (2's comp)"  force_bin_pt=on  bin_pt=0  block_type=cast
      settings: infoedit="Changes type of samples without altering their binary representation.<P><P>Hardware notes: In hardware this block costs nothing.<P><P>Example:  Suppose the input is 6 bits wide, signed, with 2 fractional bits, and the output is forced to unsigned with 0 fractional bits.  Then an input of -2.0 (1110.00 in binary 2's complement) becomes an output of 56 (111000 in binary)."  block_version=VER_STRING_GOES_HERE
  Resource Estimator : xbsIndex_r4/Resource Estimator  Tag=resEstTag  Slices=187  FFs=322  BRAMs=0  LUTs=94  IOBs=120  EBMs=0  TBUFs=0  xl_use_estimator_area=off  est_options=Estimate  xl_estimator_area=[187 322 0 94 120 0 0]  mrp_directory=D:/matlabR12/toolbox/xilinx/sysgen/bin  simulink_period=1/16  block_type=resource_estimator
      settings: AttributesFormatString=Resource\nEstimator  block_version=9.2.00
  Shift1 : xbsIndex_r4/Shift  shift_dir=Right  shift_bits=17  en=off  latency=0  precision=Full  arith_type="Signed  (2's comp)"  n_bits=8  bin_pt=2  quantization=Truncate  overflow=Wrap  dbl_ovrd=off  block_type=shift
      settings: xl_area=[0 0 0 0 0 0 0]  block_version=VER_STRING_GOES_HERE
  Shift2 : xbsIndex_r4/Shift  shift_dir=Right  shift_bits=17  en=off  latency=0  precision=Full  arith_type="Signed  (2's comp)"  n_bits=8  bin_pt=2  quantization=Truncate  overflow=Wrap  dbl_ovrd=off  block_type=shift
      settings: xl_area=[0 0 0 0 0 0 0]  block_version=VER_STRING_GOES_HERE
  Slice{1,4..6} (4 alike) : xbsIndex_r4/Slice  nbits=17  boolean_output=off  mode=Lower Bit Location + Width  bit1=18  base1=LSB of Input  bit0=0  base0=LSB of Input  dbl_ovrd=off  block_type=slice
      settings: infoedit="Extracts a given range of bits from each input sample and presents it at the output.  The output type is ordinarily unsigned with binary point at zero, but can be Boolean when the slice is one bit wide.<P><P>Hardware notes: In hardware this block costs nothing."  block_version=VER_STRING_GOES_HERE
  Slice7 : xbsIndex_r4/Slice  nbits=36  boolean_output=off  mode=Lower Bit Location + Width  bit1=18  base1=LSB of Input  bit0=0  base0=LSB of Input  dbl_ovrd=off  block_type=slice
      settings: infoedit="Extracts a given range of bits from each input sample and presents it at the output.  The output type is ordinarily unsigned with binary point at zero, but can be Boolean when the slice is one bit wide.<P><P>Hardware notes: In hardware this block costs nothing."  block_version=VER_STRING_GOES_HERE
  ab : Outport
  wires:
  Reinterpret/1 -> Convert4/1
  Convert2/1 -> Mux1/3
  Convert1/1 -> Mux1/2
  Register3/1 -> Reinterpret/1
  Concat2/1 -> Register3/1
  Register2/1 -> Concat2/1
  Register1/1 -> Concat2/2
  Delay7/1 -> Concat2/3
  Slice7/1 -> Register2/1
  Slice6/1 -> Register1/1
  Slice4/1 -> Delay7/1
  Counter/1 -> Convert5/1
  b/1 -> Delay3/1
  a/1 -> Delay1/1
  Convert/1 -> Delay8/1
  Delay9/1 -> DSP1/1
  Constant/1 -> Mux2/2
  Constant3/1 -> Mux3/2
  Constant4/1 -> Mux3/3
  Mux3/1 -> DSP1/4
  Constant1/1 -> Mux2/3
  Mux2/1 -> DSP48/3
  DSP1/1 -> Slice7/1, Slice6/1
  Delay8/1 -> DSP1/2
  Delay2/1 -> Delay5/1, Register1/2
  Delay5/1 -> Delay6/1, Register2/2
  Convert4/1 -> ab/1
  Convert3/1 -> DSP48/2
  Delay4/1 -> Mux2/1, Mux3/1, Delay2/1
  Convert5/1 -> Delay4/1, Mux1/1, Delay7/2
  Mux1/1 -> DSP48/1, Delay9/1
  Delay6/1 -> Register3/2
  Slice5/1 -> Convert1/1
  Shift1/1 -> Convert2/1
  Slice1/1 -> Convert3/1
  Shift2/1 -> Convert/1
  DSP48/1 -> Slice4/1
  DSP48/2 -> DSP1/3
  Delay1/1 -> Slice5/1, Shift1/1
  Delay3/1 -> Shift2/1, Slice1/1
